simulink model "Kinematyka"  (R2018b)
settings: Solver=FixedStepAuto  StartTime=0.0  StopTime=40.0  FixedStep=0.01  RelTol=1e-3
libraries: simulink x4
settings Model: Creator=marci  LastModifiedBy=marci

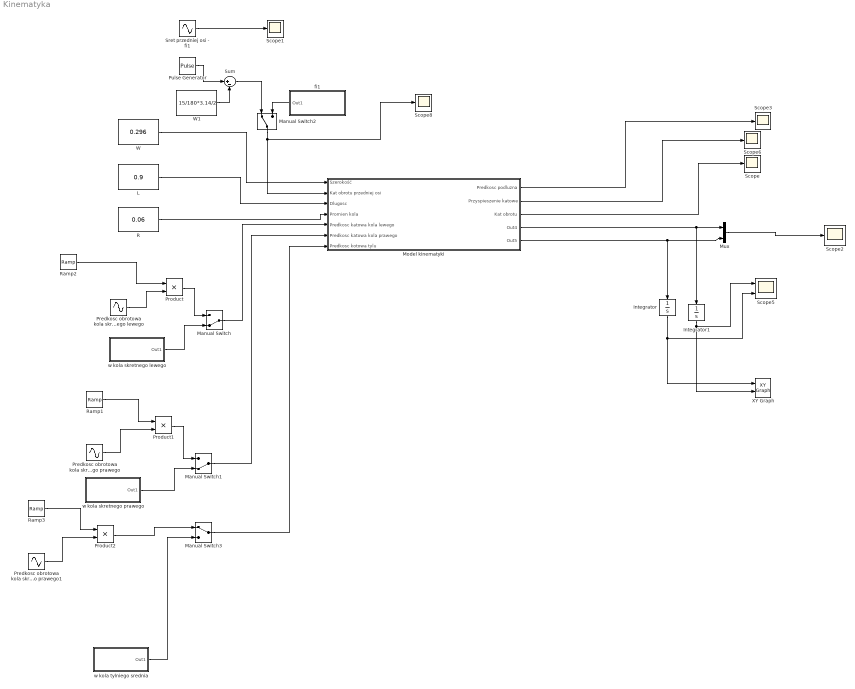
== system Kinematyka ==
  Integrator : Integrator
  Integrator1 : Integrator
  L : Constant  Value=0.9
  Manual Switch : ManualSwitch  CurrentSetting=0
  Manual Switch1 : ManualSwitch  CurrentSetting=0
  Manual Switch2 : ManualSwitch
  Manual Switch3 : ManualSwitch
  Model kinematyki : Subsystem
  Mux : Mux  Inputs=2
  Predkosc obrotowa kola skretnego lewego : Sin  Amplitude=3  Bias=5  Frequency=0.01  SampleTime=0
  Predkosc obrotowa kola skretnego prawego : Sin  Amplitude=3  Bias=5  Frequency=0.01  SampleTime=0
  Predkosc obrotowa kola skretnego prawego1 : Sin  Amplitude=3  Bias=5  Frequency=0.01  SampleTime=0
  Product : Product
  Product1 : Product
  Product2 : Product
  Pulse Generator : DiscretePulseGenerator  PulseType=Time based  Amplitude=15/180*3.14  Period=1  PulseWidth=50
  R : Constant  Value=0.06
  Ramp1 : simulink/Sources/Ramp  slope=1  start=0  InitialOutput=0
  Ramp2 : simulink/Sources/Ramp  slope=1  start=0  InitialOutput=0
  Ramp3 : simulink/Sources/Ramp  slope=1  start=0  InitialOutput=0
  Scope{,1..3,6,8} (6 alike) : Scope
  Scope5 : Scope  NumInputPorts=2
  Sret przedniej osi - fi1 : Sin  Amplitude=30/180*3.14  Frequency=0.05  SampleTime=0
  Sum : Sum  Inputs=|+-
  W : Constant  Value=0.296
  W1 : Constant  Value=15/180*3.14/2
  XY Graph : simulink/Sinks/XY Graph  xmin=-10  xmax=10  ymin=-10  ymax=10  st=-1
  fi1 : Subsystem
  w kola skretnego lewego : Subsystem
  w kola skretnego prawego : Subsystem
  w kola tylniego srednia : Subsystem
  wires:
  w kola skretnego lewego/1(Out1) -> Manual Switch/2
  w kola skretnego prawego/1(Out1) -> Manual Switch1/2
  fi1/1(Out1) -> Manual Switch2/2
  Manual Switch2/1 -> Model kinematyki/2(Kat obrotu przedniej osi), Scope8/1
  Mux/1 -> Scope2/1
  W/1 -> Model kinematyki/1(Szerokość)
  L/1 -> Model kinematyki/3(Dlugosc)
  R/1 -> Model kinematyki/4(Promien kola)
  Manual Switch/1 -> Model kinematyki/5(Predkosc katowa kola lewego)
  Manual Switch1/1 -> Model kinematyki/6(Predkosc katowa kola prawego)
  Model kinematyki/1(Predkosc podluzna) -> Scope3/1
  Model kinematyki/2(Przyspieszenie katowe) -> Scope6/1
  Model kinematyki/3(Kat obrotu) -> Scope/1
  Model kinematyki/4(Out4) -> Mux/1, Integrator1/1
  Model kinematyki/5(Out5) -> Integrator/1, Mux/2
  Pulse Generator/1 -> Sum/1
  W1/1 -> Sum/2
  Integrator/1 -> Scope5/2, XY Graph/1
  Predkosc obrotowa kola skretnego lewego/1 -> Product/2
  Ramp2/1 -> Product/1
  Product/1 -> Manual Switch/1
  Ramp1/1 -> Product1/1
  Predkosc obrotowa kola skretnego prawego/1 -> Product1/2
  Product1/1 -> Manual Switch1/1
  Sum/1 -> Manual Switch2/1
  Sret przedniej osi - fi1/1 -> Scope1/1
  w kola tylniego srednia/1(Out1) -> Manual Switch3/2
  Manual Switch3/1 -> Model kinematyki/7(Predkosc kotowa tylu)
  Ramp3/1 -> Product2/1
  Predkosc obrotowa kola skretnego prawego1/1 -> Product2/2
  Product2/1 -> Manual Switch3/1
  Integrator1/1 -> Scope5/1, XY Graph/2

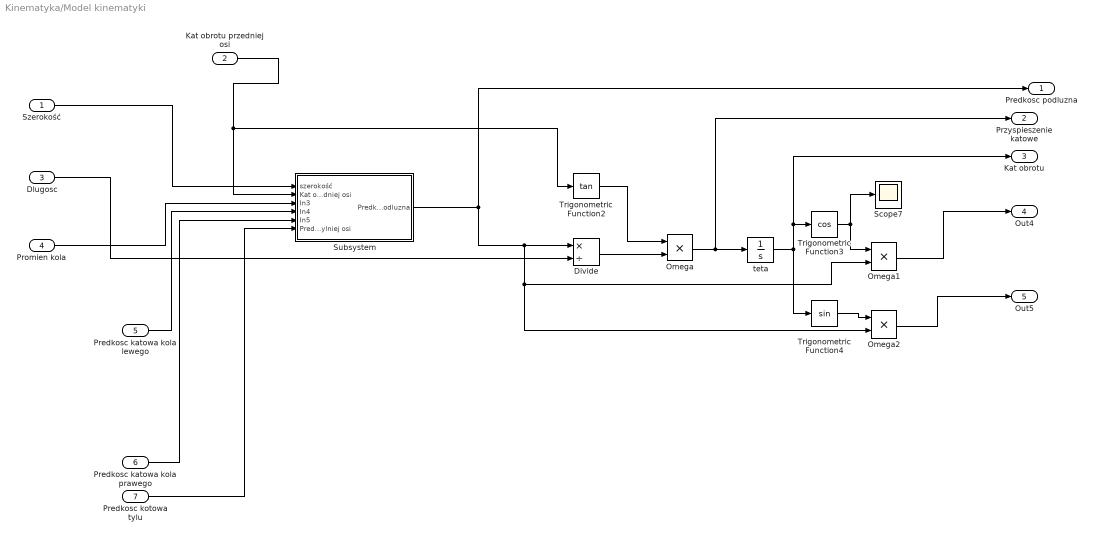
== system Kinematyka/Model kinematyki ==
  Szerokość : Inport
  Kat obrotu przedniej osi : Inport  Port=2
  Dlugosc : Inport  Port=3
  Promien kola : Inport  Port=4
  Predkosc katowa kola lewego : Inport  Port=5
  Predkosc katowa kola prawego : Inport  Port=6
  Predkosc kotowa tylu : Inport  Port=7
  Divide : Product  Inputs=*/
  Omega : Product
  Omega1 : Product
  Omega2 : Product
  Scope7 : Scope
  Subsystem : Subsystem
  Trigonometric Function2 : Trigonometry  Operator=tan
  Trigonometric Function3 : Trigonometry  Operator=cos
  Trigonometric Function4 : Trigonometry
  teta : Integrator
  Predkosc podluzna : Outport
  Przyspieszenie katowe : Outport  Port=2
  Kat obrotu : Outport  Port=3
  Out4 : Outport  Port=4
  Out5 : Outport  Port=5
  wires:
  Subsystem/1(Predkosc podluzna) -> Predkosc podluzna/1, Omega2/2, Omega1/2, Divide/1
  Divide/1 -> Omega/2
  Szerokość/1 -> Subsystem/1(szerokość)
  Kat obrotu przedniej osi/1 -> Subsystem/2(Kat obrotu przedniej osi), Trigonometric Function2/1
  Dlugosc/1 -> Divide/2
  Trigonometric Function4/1 -> Omega2/1
  Trigonometric Function2/1 -> Omega/1
  teta/1 -> Kat obrotu/1, Trigonometric Function3/1, Trigonometric Function4/1
  Trigonometric Function3/1 -> Omega1/1, Scope7/1
  Predkosc katowa kola lewego/1 -> Subsystem/4(In4)
  Omega/1 -> Przyspieszenie katowe/1, teta/1
  Omega1/1 -> Out4/1
  Promien kola/1 -> Subsystem/3(In3)
  Predkosc katowa kola prawego/1 -> Subsystem/5(In5)
  Omega2/1 -> Out5/1
  Predkosc kotowa tylu/1 -> Subsystem/6(Predkosc tylniej osi)

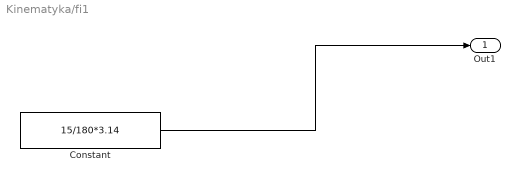
== system Kinematyka/fi1 ==
  Constant : Constant  Value=15/180*3.14
  Out1 : Outport
  wires:
  Constant/1 -> Out1/1

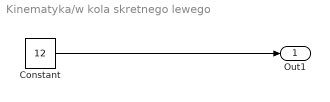
== system Kinematyka/w kola skretnego lewego ==
  Constant : Constant  Value=12
  Out1 : Outport
  wires:
  Constant/1 -> Out1/1

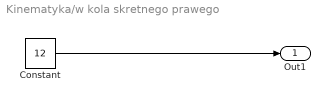
== system Kinematyka/w kola skretnego prawego ==
  Constant : Constant  Value=12
  Out1 : Outport
  wires:
  Constant/1 -> Out1/1

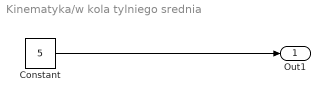
== system Kinematyka/w kola tylniego srednia ==
  Constant : Constant  Value=5
  Out1 : Outport
  wires:
  Constant/1 -> Out1/1

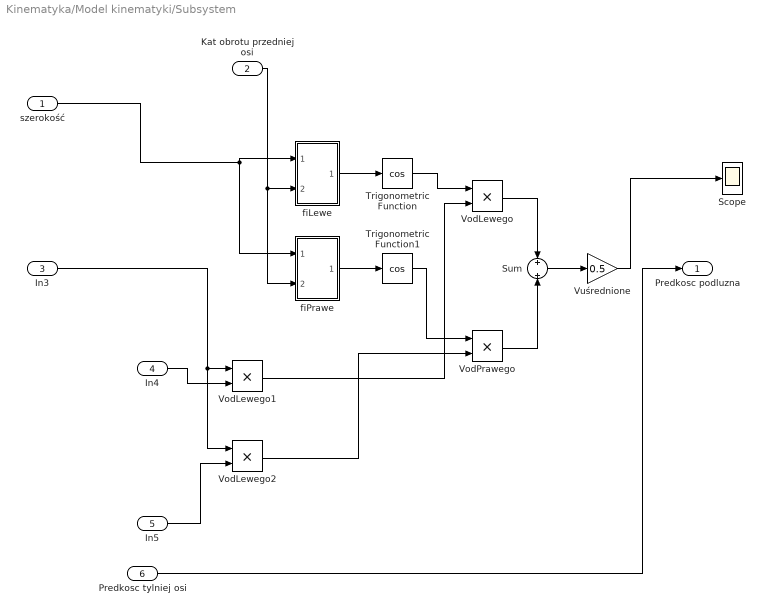
== system Kinematyka/Model kinematyki/Subsystem ==
  szerokość : Inport
  Kat obrotu przedniej osi : Inport  Port=2
  In3 : Inport  Port=3
  In4 : Inport  Port=4
  In5 : Inport  Port=5
  Predkosc tylniej osi : Inport  Port=6
  Scope : Scope
  Sum : Sum  Inputs=+||+
  Trigonometric Function : Trigonometry  Operator=cos
  Trigonometric Function1 : Trigonometry  Operator=cos
  VodLewego : Product
  VodLewego1 : Product
  VodLewego2 : Product
  VodPrawego : Product
  Vuśrednione : Gain  Gain=0.5
  fiLewe : Subsystem
  fiPrawe : Subsystem
  Predkosc podluzna : Outport
  wires:
  VodPrawego/1 -> Sum/2
  VodLewego2/1 -> VodPrawego/2
  Sum/1 -> Vuśrednione/1
  Kat obrotu przedniej osi/1 -> fiPrawe/2(In2), fiLewe/2(In2)
  Trigonometric Function1/1 -> VodPrawego/1
  szerokość/1 -> fiPrawe/1(In1), fiLewe/1(In1)
  In3/1 -> VodLewego2/1, VodLewego1/1
  fiLewe/1(Out1) -> Trigonometric Function/1
  VodLewego1/1 -> VodLewego/2
  Trigonometric Function/1 -> VodLewego/1
  VodLewego/1 -> Sum/1
  fiPrawe/1(Out1) -> Trigonometric Function1/1
  In5/1 -> VodLewego2/2
  In4/1 -> VodLewego1/2
  Predkosc tylniej osi/1 -> Predkosc podluzna/1
  Vuśrednione/1 -> Scope/1

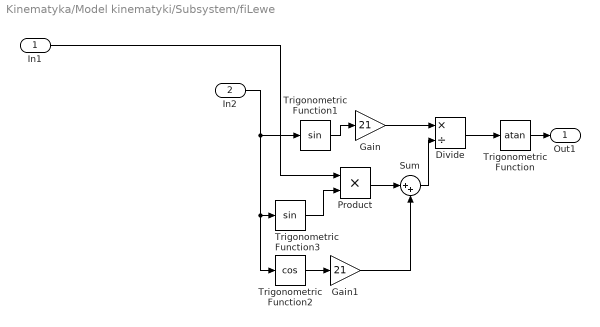
== system Kinematyka/Model kinematyki/Subsystem/fiLewe ==
  In1 : Inport
  In2 : Inport  Port=2
  Divide : Product  Inputs=*/
  Gain : Gain  Gain=21
  Gain1 : Gain  Gain=21
  Product : Product
  Sum : Sum  Inputs=|++
  Trigonometric Function : Trigonometry  Operator=atan
  Trigonometric Function1 : Trigonometry
  Trigonometric Function2 : Trigonometry  Operator=cos
  Trigonometric Function3 : Trigonometry
  Out1 : Outport
  wires:
  Gain1/1 -> Sum/2
  Gain/1 -> Divide/1
  Trigonometric Function2/1 -> Gain1/1
  In2/1 -> Trigonometric Function2/1, Trigonometric Function3/1, Trigonometric Function1/1
  Product/1 -> Sum/1
  Sum/1 -> Divide/2
  Divide/1 -> Trigonometric Function/1
  Trigonometric Function1/1 -> Gain/1
  Trigonometric Function3/1 -> Product/2
  Trigonometric Function/1 -> Out1/1
  In1/1 -> Product/1

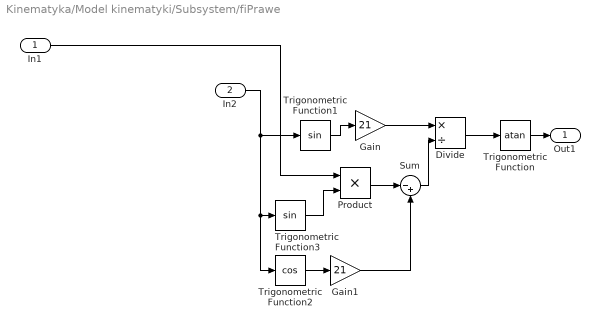
== system Kinematyka/Model kinematyki/Subsystem/fiPrawe ==
  In1 : Inport
  In2 : Inport  Port=2
  Divide : Product  Inputs=*/
  Gain : Gain  Gain=21
  Gain1 : Gain  Gain=21
  Product : Product
  Sum : Sum  Inputs=|-+
  Trigonometric Function : Trigonometry  Operator=atan
  Trigonometric Function1 : Trigonometry
  Trigonometric Function2 : Trigonometry  Operator=cos
  Trigonometric Function3 : Trigonometry
  Out1 : Outport
  wires:
  Gain1/1 -> Sum/2
  Gain/1 -> Divide/1
  Trigonometric Function2/1 -> Gain1/1
  In2/1 -> Trigonometric Function2/1, Trigonometric Function3/1, Trigonometric Function1/1
  Product/1 -> Sum/1
  Sum/1 -> Divide/2
  Divide/1 -> Trigonometric Function/1
  Trigonometric Function1/1 -> Gain/1
  Trigonometric Function3/1 -> Product/2
  Trigonometric Function/1 -> Out1/1
  In1/1 -> Product/1
